simulink model "PFC_abc_2019"  (R2023a)
settings: Solver=VariableStepAuto  StartTime=0.0  StopTime=10.0  RelTol=1e-3
undefined symbols (not defined in the file): C, Control_Udc, E, i_de, L, r, R_K_PIDf, Rch, Te, Udc_cons, w
libraries: eeTransforms x3, cstblocks x2, spsTHDLib x1
settings Model: Creator=xshi  LastModifiedBy=dougl
settings SolverCC: AlgebraicLoopSolver=TrustRegion
settings DebuggingCC: UnconnectedInputMsg=warning  UnconnectedOutputMsg=warning  UnconnectedLineMsg=warning
settings ModelReferenceCC: EnableRefExpFcnMdlSchedulingChecks=on
settings SFSimCC: CustomCodeUndefinedFunction=UseInterfaceOnly

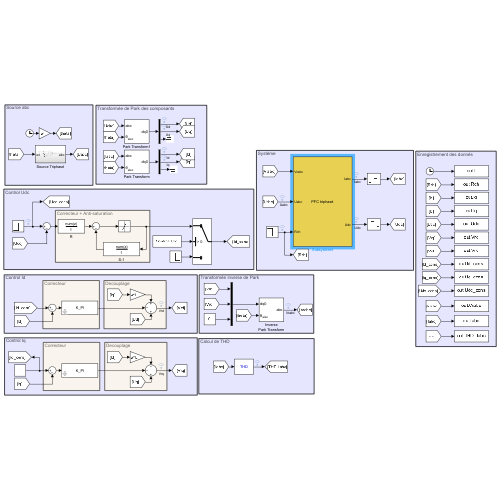
[thumbnail: Simulink's stored preview of the top-level diagram]
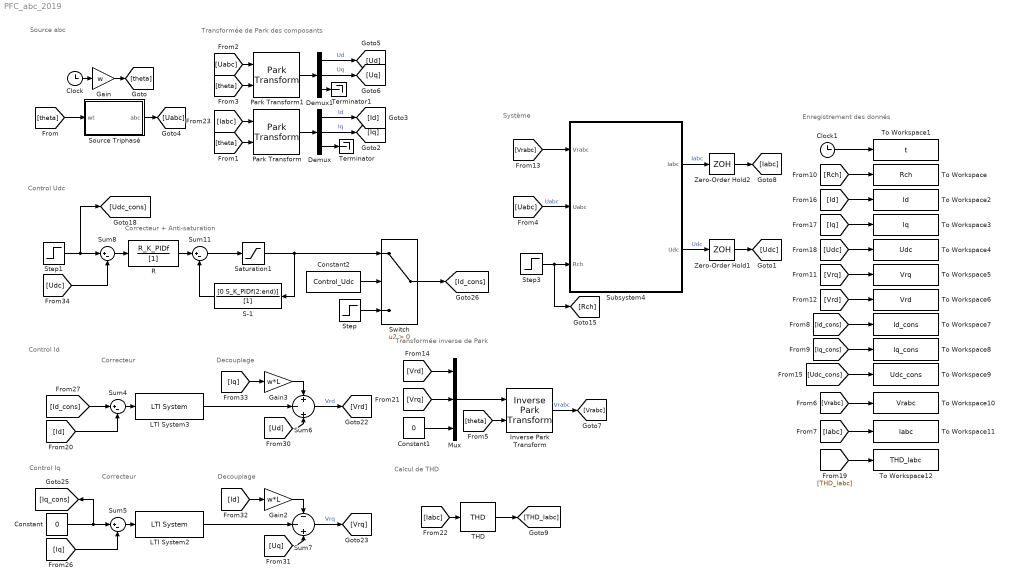
== system PFC_abc_2019 ==
  note: Enregistrement des donnés
  note: Système
  note: Calcul de THD
  note: Transformée de Park des composants
  note: Source abc
  note: Transformée inverse de Park
  note: Decouplage
  note: Correcteur
  note: Correcteur
  note: Control Id
  note: Control Udc
  note: Correcteur + Anti-saturation
  note: Decouplage
  note: Control Iq
  Clock : Clock
  Clock1 : Clock
  Constant : Constant  Value=0  SampleTime=-1
  Constant1 : Constant  Value=0
  Constant2 : Constant  Value=Control_Udc
  Demux : Demux  Outputs=3
  Demux1 : Demux  Outputs=3
  Gain : Gain  Gain=w
  Gain2 : Gain  Gain=w*L
  Gain3 : Gain  Gain=w*L
  Inverse Park Transform : eeTransforms/Inverse Park Transform  AxisAlignment=D-axis  PowerInvariant=off
      settings: LibrarySourceBlock=|
      | ee_sl_lib/Mathematical
      | Transforms/Inverse
      | Park Transform
  LTI System2 : cstblocks/LTI System  sys=K_PI  IC=[]
  LTI System3 : cstblocks/LTI System  sys=K_PI  IC=[]
  Mux : Mux  Inputs=3
  Park Transform : eeTransforms/Park Transform  AxisAlignment=D-axis  PowerInvariant=off
      settings: LibrarySourceBlock=|
      | ee_sl_lib/Mathematical
      | Transforms/Park Transform
  Park Transform1 : eeTransforms/Park Transform  AxisAlignment=D-axis  PowerInvariant=off
      settings: LibrarySourceBlock=|
      | ee_sl_lib/Mathematical
      | Transforms/Park Transform
  R : DiscreteFilter  Numerator=R_K_PIDf  Denominator=[1]  SampleTime=Te
  S-1 : DiscreteFilter  Numerator=[0 S_K_PIDf(2:end)]  Denominator=[1]  SampleTime=Te
  Saturation1 : Saturate  UpperLimit=40  LowerLimit=-40
  Source Triphasé : Subsystem
  Step : Step  Before=i_de  After=i_de/2  SampleTime=0
  Step1 : Step  Time=0  After=Udc_cons  SampleTime=0
  Step3 : Step  Time=3  Before=Rch  After=Rch/2  SampleTime=0
  Subsystem4 : Subsystem
      mask Display: disp('PFC triphasé')
  Sum{4..5,8,11} (4 alike) : Sum  Inputs=|+-
  Sum6 : Sum  Inputs=+|-|+
  Sum7 : Sum  Inputs=-|-|+
  Switch : Switch  Criteria=u2 > Threshold  SaturateOnIntegerOverflow=off  InputSameDT=off
  THD : spsTHDLib/THD  Freq=f  Ts=Te
  Terminator : Terminator
  Terminator1 : Terminator
  To Workspace : ToWorkspace  VariableName=Rch  SampleTime=Te
  To Workspace1 : ToWorkspace  VariableName=t  SampleTime=Te
  To Workspace10 : ToWorkspace  VariableName=Vrabc  SampleTime=Te
  To Workspace11 : ToWorkspace  VariableName=Iabc  SampleTime=Te
  To Workspace12 : ToWorkspace  VariableName=THD_Iabc  SampleTime=Te
  To Workspace2 : ToWorkspace  VariableName=Id  SampleTime=Te
  To Workspace3 : ToWorkspace  VariableName=Iq  SampleTime=Te
  To Workspace4 : ToWorkspace  VariableName=Udc  SampleTime=Te
  To Workspace5 : ToWorkspace  VariableName=Vrq  SampleTime=Te
  To Workspace6 : ToWorkspace  VariableName=Vrd  SampleTime=Te
  To Workspace7 : ToWorkspace  VariableName=Id_cons  SampleTime=Te
  To Workspace8 : ToWorkspace  VariableName=Iq_cons  SampleTime=Te
  To Workspace9 : ToWorkspace  VariableName=Udc_cons  SampleTime=Te
  Zero-Order Hold1 : ZeroOrderHold  SampleTime=Te
  Zero-Order Hold2 : ZeroOrderHold  SampleTime=Te
  wires:
  Clock/1 -> Gain/1
  Gain/1 -> [theta]
  [theta] -> Source Triphasé/1(wt)
  Step3/1 -> Subsystem4/3(Rch), [Rch]
  Subsystem4/2(Udc) -> Zero-Order Hold1/1  "Udc"
  [theta] -> Park Transform/2
  Park Transform/1 -> Demux/1
  Demux/2 -> [Iq]  "Iq"
  Demux/1 -> [Id]  "Id"
  Demux/3 -> Terminator/1
  Source Triphasé/1(abc) -> [Uabc]
  [Uabc] -> Park Transform1/1
  [theta] -> Park Transform1/2
  Demux1/3 -> Terminator1/1
  Demux1/1 -> [Ud]  "Ud"
  Demux1/2 -> [Uq]  "Uq"
  Park Transform1/1 -> Demux1/1
  [Uabc] -> Subsystem4/2(Uabc)  "Uabc"
  [theta] -> Inverse Park Transform/2
  Constant1/1 -> Mux/3
  Mux/1 -> Inverse Park Transform/1
  Inverse Park Transform/1 -> [Vrabc]  "Vrabc"
  [Vrq] -> To Workspace5/1
  [Udc_cons] -> To Workspace9/1
  [Id_cons] -> To Workspace7/1
  [Udc] -> To Workspace4/1
  [Id] -> To Workspace2/1
  [Iq] -> To Workspace3/1
  [Vrd] -> To Workspace6/1
  Clock1/1 -> To Workspace1/1
  [Iq_cons] -> To Workspace8/1
  [Rch] -> To Workspace/1
  Subsystem4/1(Iabc) -> Zero-Order Hold2/1  "Iabc"
  Zero-Order Hold1/1 -> [Udc]
  [Iabc] -> To Workspace11/1
  [Vrabc] -> To Workspace10/1
  Zero-Order Hold2/1 -> [Iabc]
  THD/1 -> [THD_Iabc]
  [THD_Iabc] -> To Workspace12/1
  Switch/1 -> [Id_cons]
  LTI System2/1 -> Sum7/2
  S-1/1 -> Sum11/2
  R/1 -> Sum11/1
  Sum11/1 -> Saturation1/1
  Sum7/1 -> [Vrq]  "Vrq"
  Sum8/1 -> R/1
  Saturation1/1 -> Switch/1, S-1/1
  Sum6/1 -> [Vrd]  "Vrd"
  [Iq] -> Sum5/2
  LTI System3/1 -> Sum6/2
  Gain3/1 -> Sum6/1
  Gain2/1 -> Sum7/1
  [Ud] -> Sum6/3
  [Udc] -> Sum8/2
  Sum4/1 -> LTI System3/1
  Constant2/1 -> Switch/2
  Step1/1 -> [Udc_cons], Sum8/1
  Constant/1 -> Sum5/1, [Iq_cons]
  [Id] -> Sum4/2
  [Uq] -> Sum7/3
  Sum5/1 -> LTI System2/1
  [Iq] -> Gain3/1
  [Id] -> Gain2/1
  [Id_cons] -> Sum4/1
  Step/1 -> Switch/3
  [Vrabc] -> Subsystem4/1(Vrabc)
  [Vrd] -> Mux/1
  [Vrq] -> Mux/2
  [Iabc] -> THD/1
  [Iabc] -> Park Transform/1

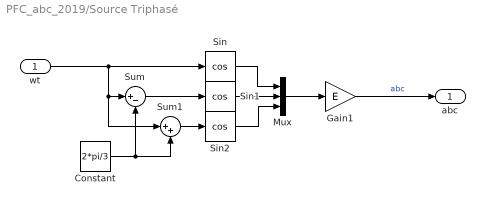
== system PFC_abc_2019/Source Triphasé ==
  wt : Inport
  Constant : Constant  Value=2*pi/3
  Gain1 : Gain  Gain=E
  Mux : Mux  Inputs=3
  Sin : Trigonometry  Operator=cos
  Sin1 : Trigonometry  Operator=cos
  Sin2 : Trigonometry  Operator=cos
  Sum : Sum  Inputs=|+-
  Sum1 : Sum  Inputs=|++
  abc : Outport
  wires:
  Constant/1 -> Sum1/2, Sum/2
  Sum1/1 -> Sin2/1
  wt/1 -> Sin/1, Sum1/1, Sum/1
  Sin/1 -> Mux/1
  Sum/1 -> Sin1/1
  Mux/1 -> Gain1/1
  Sin2/1 -> Mux/3
  Sin1/1 -> Mux/2
  Gain1/1 -> abc/1  "abc"

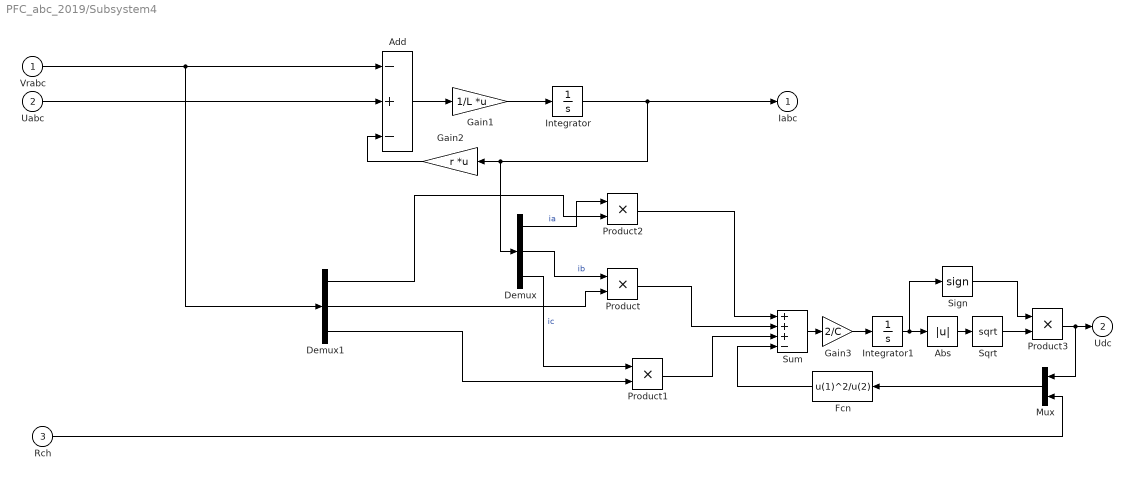
== system PFC_abc_2019/Subsystem4 ==
  Vrabc : Inport
  Uabc : Inport  Port=2
  Rch : Inport  Port=3
  Abs : Abs  SaturateOnIntegerOverflow=off
  Add : Sum  Inputs=-+-
  Demux : Demux  Outputs=3
  Demux1 : Demux  Outputs=3
  Fcn : Fcn  Expr=u(1)^2/u(2)
  Gain1 : Gain  Gain=1/L  Multiplication=Matrix(K*u)
  Gain2 : Gain  Gain=r  Multiplication=Matrix(K*u)
  Gain3 : Gain  Gain=2/C
  Integrator : Integrator
  Integrator1 : Integrator  InitialCondition=400^2
  Mux : Mux  Inputs=2
  Product{,1..3} (4 alike) : Product
  Sign : Signum
  Sqrt : Sqrt
  Sum : Sum  Inputs=+++-
  Iabc : Outport  InitialOutput=0
  Udc : Outport  Port=2  InitialOutput=0
  wires:
  Vrabc/1 -> Demux1/1, Add/1
  Add/1 -> Gain1/1
  Gain1/1 -> Integrator/1
  Gain2/1 -> Add/3
  Uabc/1 -> Add/2
  Integrator/1 -> Demux/1, Gain2/1, Iabc/1
  Demux/3 -> Product1/1  "ic"
  Sum/1 -> Gain3/1
  Demux1/3 -> Product1/2
  Demux/2 -> Product/1  "ib"
  Demux1/2 -> Product/2
  Rch/1 -> Mux/2
  Mux/1 -> Fcn/1
  Demux1/1 -> Product2/2
  Demux/1 -> Product2/1  "ia"
  Fcn/1 -> Sum/4
  Product1/1 -> Sum/3
  Product/1 -> Sum/2
  Product2/1 -> Sum/1
  Abs/1 -> Sqrt/1
  Integrator1/1 -> Sign/1, Abs/1
  Gain3/1 -> Integrator1/1
  Sqrt/1 -> Product3/2
  Sign/1 -> Product3/1
  Product3/1 -> Mux/1, Udc/1
